simulink model "FailureExample"  (Simulink 7.8)
settings: Solver=ode45  StartTime=0.0  StopTime=6  RelTol=1e-3
settings Model: Creator=lind_fr  LastModifiedBy=lind_fr

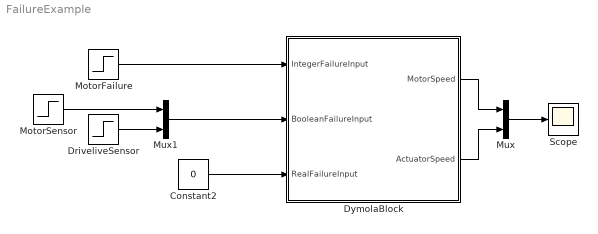
== system FailureExample ==
  Constant2 : Constant  Value=0
  DriveliveSensor : Step  Time=5  SampleTime=0
  DymolaBlock : Subsystem  Tag=25-Jul-2012 16:53:41#8147
      settings: CopyFcn=newDymolaGui('25-Jul-2012 16:53:41#8147','Copy');  DeleteFcn=if exist('newDymolaGui') newDymolaGui('FailureExample/DymolaBlock','Delete'); end;  NameChangeFcn=newDymolaGui('25-Jul-2012 16:53:41#8147','Copy');  OpenFcn=newDymolaGui('FailureExample/DymolaBlock','Init');
      mask Description:
      | Dymola block.
      | A dymola block allows acausal physical modeling.
      | See Dymola manual for usage.
      mask Display: image(reshape([1;1;1;1;1;1;1;1;1;1;1;1;1;1;1;1;1;1;1;1;1;1;0;0;0;0;0;0;0;0;0;0;1;1;1;1;1;1;1;1;0;1;1;1;1;1;1;1;1;0;1;1;1;1;1;0;0;0;0;0;0;0;1;1;0;0;0;0;0;0;0;1;1;0;0;0;0;0;0;0;1;1;0;0;0;0;0;0;0;1;1;0;0;0;0;0;0;0;1;1;0;0;0;0;0;0;0;1;1;0;0;0;0;0;0;0;1;1;0;0;0;0;0;0;0;1;1;0;0;0;0;0;0;0;1;1;0;0;0;0;0;0;0;1;1;0;0;0;0;0;0;0;1;1;0;0;0;0;0;0;0;1;1;0;0;0;0;0;0;0;1;1;0;0;0;0;0;0;0;1;1;0;0;0;0;0;0;0;1;1;0;0;0;0;0;0;0;1;1;0;0;0;0;0;0;0;1;1;0;0;0;0;0;0;0;1;1;0;0;0;0;0;0;0;1;1;0;0;0;0;0;0;0;1;1;0;0;0;0;0;0;0;1;1;0;0;0;0;0;0;0;1;1;0;0;0;0;0;0;0;1;1;0;0;0;0;0;0;0;1;1;1;1;1;0;1;1;1;1;1;1;1;1;0;1;1;1;1;1;1;1;1;0;0;0;0;0;0;0;0;0;0;1;1;1;1;1;1;1;1;1;1;1;1;1;1;1;1;1;1;1;1;1;1;1;1;1;1;1;1;1;1;1;1;1;1;1;1;1;1;1;1;1;1;1;1;0;0;0;0;0;0;0;0;0;0;1;1;1;1;1;1;1;1;0;1;1;1;1;1;1;1;1;0;1;1;1;1;1;0;0;0;0;0;0;0;1;1;0;0;0;0;0;0;0;1;1;0;0;0;0;0;0;0;1;1;0;0;0;0;0;0;0;1;1;0;0;0;0;0;0;0;1;1;0;0;0;0;0;0;0;1;1;0;0;0;0;0;0;0;1;1;0;0;0;0;0;0;0;1;1;0;0;0;0;0;0;0;1;1;0;0;0;0;0;0;0;1;1;0;0;0;0;0;0;0;1;1;0;0;0;0;0;0;0;1;1;0;0;0;0;0;0;0;1;1;0;0;0;0;0;0;0;1;1;0;0;0;0;0;0;0;1;1;0;0;0;0;0;0;0;1;1;0;0;0;0;0;0;0;1;1;0;0;0;0;0;0;0;1;1;0;0;0;0;0;0;0;1;1;0;0;0;0;0;0;0;1;1;0;0;0;0;0;0;0;1;1;0;0;0;0;0;0;0;1;1;0;0;0;0;0;0;0;1;1;0;0;0;0;0;0;0;1;1;1;1;1;0;1;1;1;1;1;1;1;1;0;1;1;1;1;1;1;1;1;0;0;0;0;0;0;0;0;0;0;1;1;1;1;1;1;1;1;1;1;1;1;1;1;1;1;1;1;1;1;1;1;1;1;1;1;1;1;1;1;1;1;1;1;1;1;1;1;1;1;1;1;1;1;0;0;0;0;0;0;0;0;0;0;1;1;1;1;1;1;1;1;0;1;1;1;1;1;1;1;1;0;1;1;1;1;1;0;0;0;0;0;0;0;1;1;0;0;0;0;0;0;0;1;1;0;1;1;1;1;1;0;1;1;0;1;1;1;1;1;0;1;1;0;1;1;1;1;1;0;1;1;0;1;1;1;1;1;0;1;1;0;1;1;1;1;1;0;1;1;0;1;1;1;1;1;0;1;1;0;1;1;1;1;1;0;1;1;0;1;1;1;1;1;0;1;1;0;1;1;1;1;1;0;1;1;0;1;1;1;1;1;0;1;1;0;1;1;1;1;1;0;1;1;0;1;1;1;1;1;0;1;1;0;1;1;1;1;1;0;1;1;0;1;1;1;1;1;0;1;1;0;1;1;1;1;1;0;1;1;0;1;1;1;1;1;0;1;1;0;1;1;1;1;1;0;1;1;0;1;1;1;1;1;0;1;1;0;1;1;1;1;1;0;1;1;0;1;1;1;1;1;0;1;1;0;0;0;0;0;0;0;1;1;0;0;0;0;0;0;0;1;1;1;1;1;0;1;1;1;1;1;1;1;1;0;1;1;1;1;1;1;1;1;0;0;0;0;0;0;0;0;0;0;1;1;1;1;1;1;1;1;1;1;1;1;1;1;1;1;1;1;1;1;1;1],18,18,3),[.2,.2,.6,.6])
  MotorFailure : Step  Time=.5  Before=1  After=2  SampleTime=0
  MotorSensor : Step  Time=3  SampleTime=0
  Mux : Mux  Inputs=2
  Mux1 : Mux  Inputs=2
  Scope : Scope
  wires:
  Mux/1 -> Scope/1
  Constant2/1 -> DymolaBlock/3(RealFailureInput)
  DymolaBlock/1(MotorSpeed) -> Mux/1
  DymolaBlock/2(ActuatorSpeed) -> Mux/2
  MotorSensor/1 -> Mux1/1
  DriveliveSensor/1 -> Mux1/2
  MotorFailure/1 -> DymolaBlock/1(IntegerFailureInput)
  Mux1/1 -> DymolaBlock/2(BooleanFailureInput)

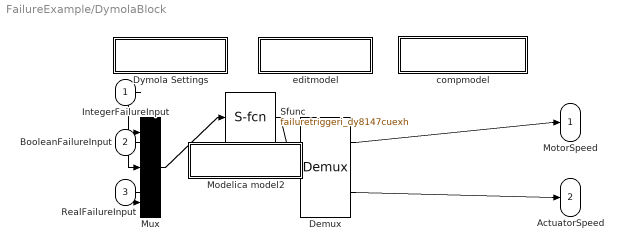
== system FailureExample/DymolaBlock ==
  IntegerFailureInput : Inport
  BooleanFailureInput : Inport  Port=2
  RealFailureInput : Inport  Port=3
  Demux : Demux  Outputs=[1;1]
  Dymola Settings : Subsystem  mask{ModelName=FailureTriggering.Examples.MotorExample.ActuatorExternalFault, MoFileName=Z:/Actuation 2015/WP3_4/FailureTriggering/Code/FailureTriggering.mo, dSpace=, BusConnector=[], ResultFile=[], ResultFileOnline=[], ResultDt=[], Libs=:, bigobj=[], ImportFolder=[], guimode=[], ModelName2=[], forRuntime=[], MEXLoad=[]}
      mask prompts: ModelName "Name of Dymola model"; MoFileName "File Name (including .mo)"; ResultFile "Create Result"; ResultFileOnline "Load result"; ResultDt "Result min dt"; Libs "Used Libraries"; bigobj "Compiler flag /bigobj"; ImportFolder "Import folder"; guimode "GUI mode flag"; ModelName2 "Model name for import mode"; forRuntime "Runtime export"; MEXLoad "Compiled S-function"
      mask Display: disp('Dymola Settings');
  Modelica model2 : Subsystem
      mask Display: disp('Change parameters');
  Mux : Mux  Inputs=[1;2;1]
  Sfunc : S-Function  Tag=8147cuexh  FunctionName=failuretriggeri_dy8147cuexh  Parameters=[quadraticSpeedDependentTo1;quadraticSpeedDependentTo2;motor_bokenKt_k;motor_halfBrokenKt_k;motor_motorInertia_J;motor_kt_selection_allowO6;motor_kt_selection_outOfR7;motor_healthyKt_k;motor_speedSensor_fault_l9;motor_speedSensor_externa10;motor_speedSensor_externa11;motor_motorTorqueReferenc12;motor_motorKtFailure_faul13;motor_motorKtFailure_exte14;motor_motorKtFailure_exte15;driveline_DriveFriction_f16;driveline_DriveFriction_e17;driveline_DriveFriction_e18;driveline_DrivelineDiscon19;driveline_booleanToReal_r20;driveline_booleanToReal_r21;driveline_Driveline_Break22;driveline_Driveline_Break23;driveline_Driveline_Break24;driveline_Driveline_Break25;driveline_Driveline_Break26;driveline_inertia_J;driveline_brake_mue_pos;driveline_brake_peak;driveline_brake_cgeo;driveline_brake_fn_max;driveline_brake_w_small;driveline_idealGear_ratio;driveline_SpeedSensor_fau34;driveline_SpeedSensor_ext35;driveline_SpeedSensor_ext36],[quadraticSpeedDependentTo37;driveline_Driveline_Break38;driveline_Driveline_Break39;driveline_inertia_w]  PortCounts=[1;1]  EnableBusSupport=off  mask{quadraticSpeedDependentTo1=-0.1, quadraticSpeedDependentTo2=1, motor_bokenKt_k=0, motor_halfBrokenKt_k=0.5, motor_motorInertia_J=0.001, motor_kt_selection_allowO6=0, motor_kt_selection_outOfR7=10000000000, motor_healthyKt_k=1, motor_speedSensor_fault_l9=0, motor_speedSensor_externa10=1, motor_speedSensor_externa11=1, motor_motorTorqueReferenc12=1, motor_motorKtFailure_faul13=1, motor_motorKtFailure_exte14=1, motor_motorKtFailure_exte15=1, driveline_DriveFriction_f16=0, driveline_DriveFriction_e17=1, driveline_DriveFriction_e18=1, driveline_DrivelineDiscon19=0, driveline_booleanToReal_r20=0, driveline_booleanToReal_r21=1, driveline_Driveline_Break22=[0; 0.5], driveline_Driveline_Break23=1, driveline_Driveline_Break24=1, driveline_Driveline_Break25=100, driveline_Driveline_Break26=10000000000, driveline_inertia_J=0.001, driveline_brake_mue_pos=[0; 0.5], driveline_brake_peak=1, driveline_brake_cgeo=1, driveline_brake_fn_max=100, driveline_brake_w_small=10000000000, driveline_idealGear_ratio=2, driveline_SpeedSensor_fau34=0, driveline_SpeedSensor_ext35=2, driveline_SpeedSensor_ext36=1, quadraticSpeedDependentTo37=0, driveline_Driveline_Break38=0, driveline_Driveline_Break39=0, driveline_inertia_w=0}
      mask prompts: quadraticSpeedDependentTo1 "quadraticSpeedDependentTorque.tau_nominal"; quadraticSpeedDependentTo2 "quadraticSpeedDependentTorque.w_nominal"; motor_bokenKt_k "motor.bokenKt.k"; motor_halfBrokenKt_k "motor.halfBrokenKt.k"; motor_motorInertia_J "motor.motorInertia.J"; motor_kt_selection_allowO6 "motor.kt_selection.allowOutOfRange"; motor_kt_selection_outOfR7 "motor.kt_selection.outOfRangeValue"; motor_healthyKt_k "motor.healthyKt.k"; motor_speedSensor_fault_l9 "motor.speedSensor.fault_local"; motor_speedSensor_externa10 "motor.speedSensor.externalFault.faultIndex"; motor_speedSensor_externa11 "motor.speedSensor.externalFault.externalFaultOn"; motor_motorTorqueReferenc12 "motor.motorTorqueReference.k"; motor_motorKtFailure_faul13 "motor.motorKtFailure.fault_local"; motor_motorKtFailure_exte14 "motor.motorKtFailure.externalFault.faultIndex"; motor_motorKtFailure_exte15 "motor.motorKtFailure.externalFault.externalFaultOn"; driveline_DriveFriction_f16 "driveline.DriveFriction.fault_local"; driveline_DriveFriction_e17 "driveline.DriveFriction.externalFault.faultIndex"; driveline_DriveFriction_e18 "driveline.DriveFriction.externalFault.externalFaultOn"; driveline_DrivelineDiscon19 "driveline.DrivelineDisconnect.k"; driveline_booleanToReal_r20 "driveline.booleanToReal.realTrue"; driveline_booleanToReal_r21 "driveline.booleanToReal.realFalse"; driveline_Driveline_Break22 "driveline.Driveline_Break.mue_pos"; driveline_Driveline_Break23 "driveline.Driveline_Break.peak"; driveline_Driveline_Break24 "driveline.Driveline_Break.cgeo"; driveline_Driveline_Break25 "driveline.Driveline_Break.fn_max"; driveline_Driveline_Break26 "driveline.Driveline_Break.w_small"; driveline_inertia_J "driveline.inertia.J"; driveline_brake_mue_pos "driveline.brake.mue_pos"; driveline_brake_peak "driveline.brake.peak"; driveline_brake_cgeo "driveline.brake.cgeo"; driveline_brake_fn_max "driveline.brake.fn_max"; driveline_brake_w_small "driveline.brake.w_small"; driveline_idealGear_ratio "driveline.idealGear.ratio"; driveline_SpeedSensor_fau34 "driveline.SpeedSensor.fault_local"; driveline_SpeedSensor_ext35 "driveline.SpeedSensor.externalFault.faultIndex"; driveline_SpeedSensor_ext36 "driveline.SpeedSensor.externalFault.externalFaultOn"; quadraticSpeedDependentTo37 "quadraticSpeedDependentTorque.phi"; driveline_Driveline_Break38 "driveline.Driveline_Break.phi_rel"; driveline_Driveline_Break39 "driveline.Driveline_Break.w_rel"; driveline_inertia_w "driveline.inertia.w"
      mask Display: image(imread('Dymola.bmp'))
  compmodel : Subsystem
      settings: OpenFcn=compileModelica('FailureExample/DymolaBlock');
      mask Display: disp('Compile Modelica model');
  editmodel : Subsystem
      settings: OpenFcn=editModelica('FailureExample/DymolaBlock');
      mask Display: disp('Edit Modelica model');
  MotorSpeed : Outport
  ActuatorSpeed : Outport  Port=2
  wires:
  Sfunc/1 -> Demux/1
  Demux/1 -> MotorSpeed/1
  Demux/2 -> ActuatorSpeed/1
  Mux/1 -> Sfunc/1
  IntegerFailureInput/1 -> Mux/1
  BooleanFailureInput/1 -> Mux/2
  RealFailureInput/1 -> Mux/3

== system FailureExample/DymolaBlock/Dymola Settings ==

== system FailureExample/DymolaBlock/Modelica model2 ==

== system FailureExample/DymolaBlock/compmodel ==

== system FailureExample/DymolaBlock/editmodel ==
